simulink model "regulator"  (R2021a)
settings: Solver=VariableStepAuto  StartTime=0.0  StopTime=10.0  RelTol=1e-3
values from neighbouring files (symbols this model uses):
  k = place(sysestc.A, sysestc.B, new_pole)    [PolePlacement.m]    (also in PolePlacement_Controller_script.m = place(A, B, new_pole); ppObs.m)
  Kr = 1/Kdc(1)    [PolePlacement.m]    (also in PolePlacement_Controller_script.m; ppObs.m)
  L = place(sysestc.A',sysestc.C', 10*new_pole)'    [PolePlacement.m]    (also in PolePlacement_Controller_script.m; ppObs.m)
  sysestc = d2c(sysest)    [PolePlacement.m]    (also in PolePlacement_Controller_script.m; ppObs.m)
undefined symbols (not defined in the file or in its folder): dem, Gp, Kp, num, sigbuilder_block, Ti
libraries: cstblocks x2
settings Model: Creator=jesuc  LastModifiedBy=arco

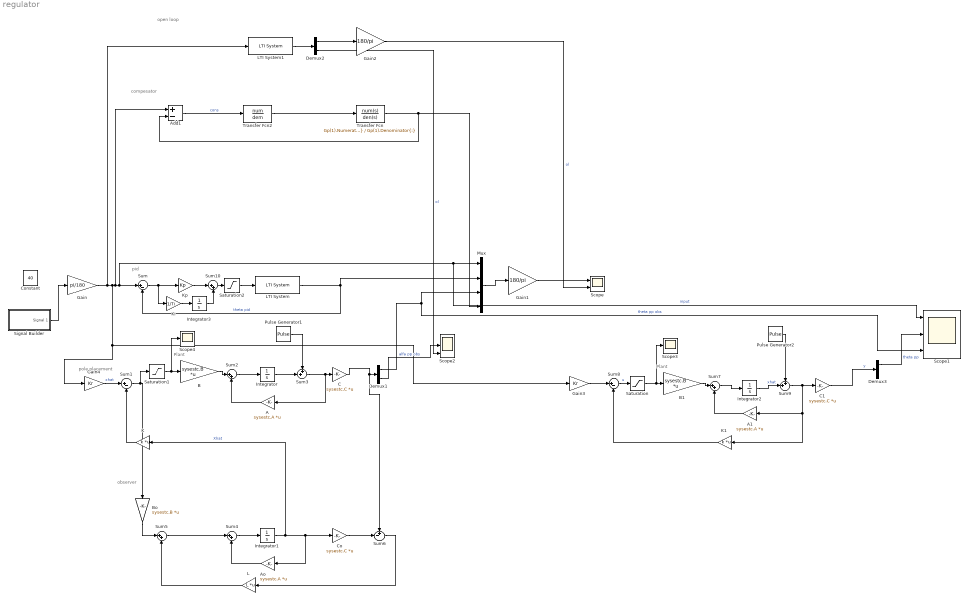
== system regulator ==
  note: pid
  note: pole placement
  note: observer
  note: compesator
  note: open loop
  note: Plant
  note: Plant
  A : Gain  Gain=sysestc.A  Multiplication=Matrix(K*u)
  A1 : Gain  Gain=sysestc.A  Multiplication=Matrix(K*u)
  Add1 : Sum  Inputs=+-
  Ao : Gain  Gain=sysestc.A  Multiplication=Matrix(K*u)
  B : Gain  Gain=sysestc.B  Multiplication=Matrix(K*u)
  B1 : Gain  Gain=sysestc.B  Multiplication=Matrix(K*u)
  Bo : Gain  Gain=sysestc.B  Multiplication=Matrix(K*u)
  C : Gain  Gain=sysestc.C  Multiplication=Matrix(K*u)
  C1 : Gain  Gain=sysestc.C  Multiplication=Matrix(K*u)
  Co : Gain  Gain=sysestc.C  Multiplication=Matrix(K*u)
  Constant : Constant  Value=40
  Demux1 : Demux  Outputs=2
  Demux2 : Demux  Outputs=2
  Demux3 : Demux  Outputs=2
  Gain : Gain  Gain=pi/180
  Gain1 : Gain  Gain=180/pi
  Gain2 : Gain  Gain=180/pi
  Gain3 : Gain  Gain=Kr
  Gain4 : Gain  Gain=Kr
  Integrator{,1..3} (4 alike) : Integrator
  K : Gain  Gain=k  Multiplication=Matrix(K*u)
  K1 : Gain  Gain=k  Multiplication=Matrix(K*u)
  Ki : Gain  Gain=1/Ti
  Kp : Gain  Gain=Kp
  L : Gain  Gain=L  Multiplication=Matrix(K*u)
  LTI System : cstblocks/LTI System  sys=Gp(1)  IC=[]
  LTI System1 : cstblocks/LTI System  sys=tf(sysestc)  IC=[]
  Mux : Mux
  Pulse Generator1 : DiscretePulseGenerator  PulseType=Time based  Amplitude=0  Period=1.5  PulseWidth=5
  Pulse Generator2 : DiscretePulseGenerator  PulseType=Time based  Amplitude=.2  Period=1.5  PulseWidth=5
  Saturation : Saturate  UpperLimit=5  LowerLimit=-5
  Saturation1 : Saturate  UpperLimit=5  LowerLimit=-5
  Saturation2 : Saturate  UpperLimit=5  LowerLimit=-5
  Scope : Scope  NumInputPorts=2
  Scope1 : Scope  NumInputPorts=3
  Scope2 : Scope  NumInputPorts=3
  Scope3 : Scope
  Scope4 : Scope
  Signal Builder : Subsystem  Tag=STV Subsys  LoadFcn=sigbuilder_block('load');  StartFcn=sigbuilder_block('start');  StopFcn=sigbuilder_block('stop');  ClipboardFcn=sigbuilder_block('clipboard');  mask(Sigbuilder block){tuvar=[0:10]}
      mask help: Simulink:masks:SigbuilderBlock_MD
      mask init:
      | if ~strcmp(get_param(bdroot(gcbh),'SimulationStatus'),'stopped') tuvar = sigbuilder_block('maskInit'); end
      settings: CopyFcn=sigbuilder_block('copy');  DeleteFcn=sigbuilder_block('delete');  ModelCloseFcn=sigbuilder_block('modelClose');  PreSaveFcn=sigbuilder_block('preSave');  PauseFcn=sigbuilder_block('pause');  ContinueFcn=sigbuilder_block('continue');  NameChangeFcn=sigbuilder_block('namechange');  OpenFcn=sigbuilder_block('open',[437.6 199.2 550.4 400 ]);  CloseFcn=sigbuilder_block('close');
      mask Display: plot(0, 0, 100, 100,[2, 2, 32, 32, 2], [68, 8, 8, 68, 68],[32, 2], [38, 38], [32, 19, 2],[53, 60, 44], [32, 17, 17, 2],[16, 16, 31, 31]);txt = getActiveGroup(gcbh);text(2, 100, txt,'verticalAlignment', 'top');
  Sum : Sum  Inputs=|+-
  Sum1 : Sum  Inputs=|+-
  Sum{2,4..5,7,10} (5 alike) : Sum  Inputs=|++
  Sum3 : Sum  Inputs=++|
  Sum6 : Sum  Inputs=+-|
  Sum8 : Sum  Inputs=|+-
  Sum9 : Sum  Inputs=++|
  Transfer Fcn : TransferFcn  Numerator=Gp(1).Numerator{:}  Denominator=Gp(1).Denominator{:}
  Transfer Fcn2 : TransferFcn  Numerator=num  Denominator=dem
  wires:
  LTI System/1 -> Mux/2, Sum/2  "theta pid"
  B/1 -> Sum2/1
  Sum2/1 -> Integrator/1
  A/1 -> Sum2/2
  K/1 -> Sum1/2
  Demux1/1 -> Scope1/3, Mux/3  "theta pp obs"
  Demux1/2 -> Scope2/2  "alfa pp obs"
  Gain1/1 -> Scope/1
  Mux/1 -> Gain1/1
  LTI System1/1 -> Demux2/1
  Demux2/1 -> Gain2/1
  Gain2/1 -> Scope/2  "ol"
  Demux2/2 -> Scope2/3  "ol"
  C1/1 -> Demux3/1  "y"
  Demux3/1 -> Scope1/2  "theta pp"
  Integrator1/1 -> K/1, Ao/1, Co/1  "Xhat"
  L/1 -> Sum5/2
  Sum6/1 -> L/1
  Ao/1 -> Sum4/2
  Co/1 -> Sum6/2
  Sum5/1 -> Sum4/1
  Sum4/1 -> Integrator1/1
  Bo/1 -> Sum5/1
  B1/1 -> Sum7/1
  Sum7/1 -> Integrator2/1
  A1/1 -> Sum7/2
  K1/1 -> Sum8/2
  Sum8/1 -> Saturation/1  "u"
  Gain3/1 -> Sum8/1
  Gain4/1 -> Sum1/1  "xhat"
  Sum1/1 -> Saturation1/1, Bo/1
  Saturation/1 -> Scope3/1, B1/1
  Pulse Generator1/1 -> Sum3/1
  C/1 -> Sum6/1, Demux1/1
  Integrator2/1 -> Sum9/2  "xhat"
  Pulse Generator2/1 -> Sum9/1
  Sum9/1 -> K1/1, A1/1, C1/1
  Integrator/1 -> Sum3/2
  Sum3/1 -> A/1, C/1
  Saturation1/1 -> Scope4/1, B/1
  Transfer Fcn2/1 -> Transfer Fcn/1
  Transfer Fcn/1 -> Add1/2, Mux/4
  Add1/1 -> Transfer Fcn2/1  "cons"
  Saturation2/1 -> LTI System/1
  Integrator3/1 -> Sum10/2
  Sum10/1 -> Saturation2/1
  Signal Builder/1(Signal 1) -> Gain/1
  Kp/1 -> Sum10/1
  Sum/1 -> Ki/1, Kp/1
  Ki/1 -> Integrator3/1
  Gain/1 -> LTI System1/1, Gain4/1, Gain3/1, Add1/1, Scope1/1, Mux/1, Sum/1  "input"

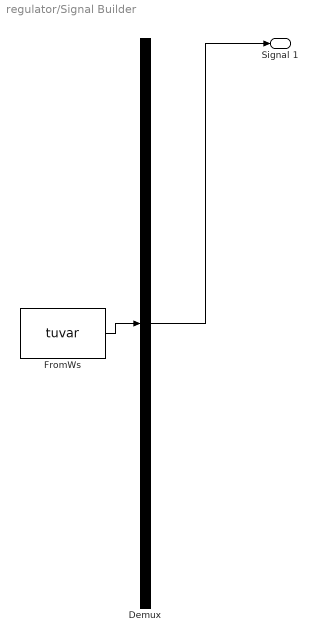
== system regulator/Signal Builder ==
  Demux : Demux  Tag=STV Demux  Outputs=1
      settings: DisplayOption=none
  FromWs : FromWorkspace  Tag=STV FromWs  VariableName=tuvar
      SigBuilderData=|
      | common.afterFinalStr = 'Extrapolate'
      | common.sampleTime = 0
      | dataSet.timeRange = [0 10]
      | dataSet.name = 'Group 1'
      | sbobj.Groups.Name = 'Group 1'
      | sbobj.Groups.Signals.Name = 'Signal 1'
      | sbobj.Groups.Signals.XData = [0 1 1 3 3 5 5 7 7 8.5 8.5 10]
      | sbobj.Groups.Signals.YData = [0.005 0.005 40 40 15 15 -30 -30 0 0 23 23]
  Signal 1 : Outport  Tag=STV Outport
  wires:
  Demux/1 -> Signal 1/1
  FromWs/1 -> Demux/1
